simulink library "csu_rtd_translational_dynamics_lib"  (R2014b)
settings: Solver=ode45  SolverMode=SingleTasking  StartTime=0.0  StopTime=10.0  RelTol=1e-3
libraries: util_info_lib x2, util_quat_lib x2, util_integrator_lib x1
settings Model: ExtModeAutoUpdateStatusClock=off  Creator=daniloviazzo  LastModifiedBy=mstewart

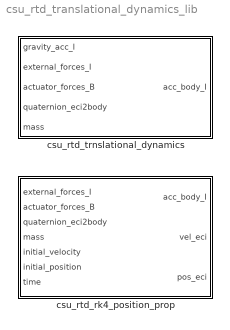
== system csu_rtd_translational_dynamics_lib ==
  csu_rtd_rk4_position_prop : Subsystem
  csu_rtd_trnslational_dynamics : Subsystem

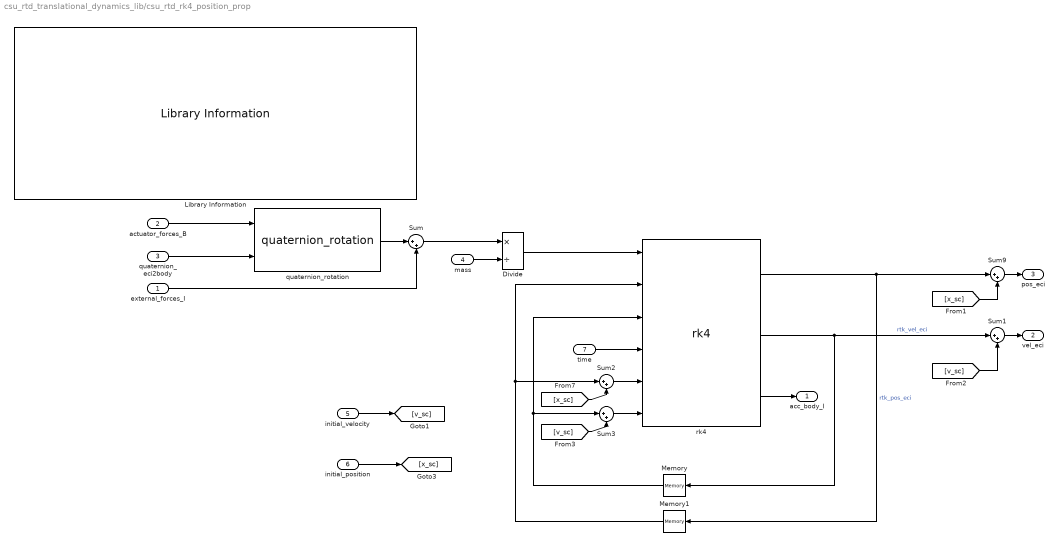
== system csu_rtd_translational_dynamics_lib/csu_rtd_rk4_position_prop ==
  external_forces_I : Inport
  actuator_forces_B : Inport  Port=2
  quaternion_eci2body : Inport  Port=3
  mass : Inport  Port=4
  initial_velocity : Inport  Port=5
  initial_position : Inport  Port=6
  time : Inport  Port=7
  Divide : Product  Inputs=*/
  Library Information : util_info_lib/Library Information  owner='NONE'
  Memory : Memory  InheritSampleTime=on
  Memory1 : Memory  InheritSampleTime=on
  Sum{,1..3,9} (5 alike) : Sum  Inputs=|++
  quaternion_rotation : util_quat_lib/quaternion_rotation  SystemSampleTime=-1
  rk4 : util_integrator_lib/rk4  DT=sim_time_step_size
  acc_body_I : Outport
  vel_eci : Outport  Port=2
  pos_eci : Outport  Port=3
  wires:
  [v_sc] -> Sum3/2
  initial_velocity/1 -> [v_sc]
  [v_sc] -> Sum1/2
  Sum3/1 -> rk4/6
  initial_position/1 -> [x_sc]
  [x_sc] -> Sum2/2
  Sum2/1 -> rk4/5
  [x_sc] -> Sum9/2
  Sum1/1 -> vel_eci/1
  Sum9/1 -> pos_eci/1
  Memory1/1 -> Sum2/1, rk4/2
  Memory/1 -> Sum3/1, rk4/3
  rk4/1 -> Sum9/1, Memory1/1  "rtk_pos_eci"
  time/1 -> rk4/4
  rk4/2 -> Sum1/1, Memory/1  "rtk_vel_eci"
  rk4/3 -> acc_body_I/1
  mass/1 -> Divide/2
  Sum/1 -> Divide/1
  external_forces_I/1 -> Sum/2
  quaternion_rotation/1 -> Sum/1
  quaternion_eci2body/1 -> quaternion_rotation/2
  Divide/1 -> rk4/1
  actuator_forces_B/1 -> quaternion_rotation/1

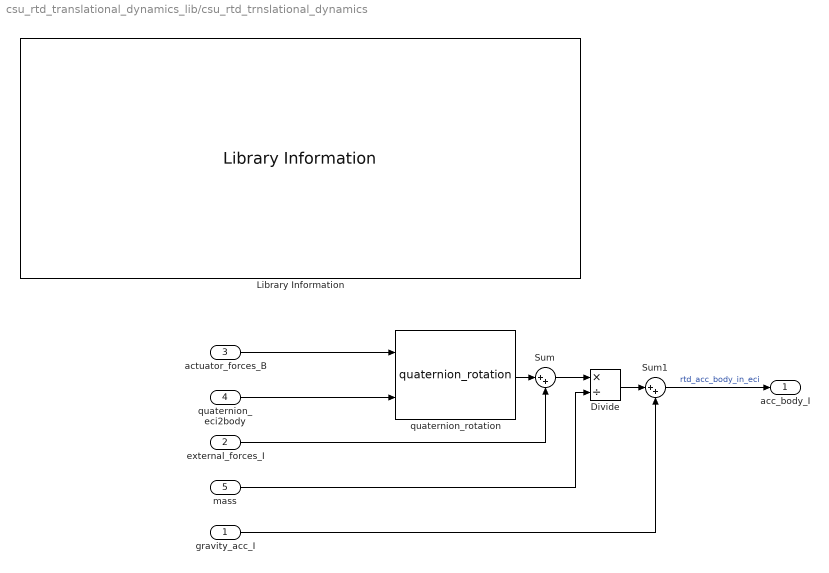
== system csu_rtd_translational_dynamics_lib/csu_rtd_trnslational_dynamics ==
  gravity_acc_I : Inport
  external_forces_I : Inport  Port=2
  actuator_forces_B : Inport  Port=3
  quaternion_eci2body : Inport  Port=4
  mass : Inport  Port=5
  Divide : Product  Inputs=*/
  Library Information : util_info_lib/Library Information  owner='NONE'
  Sum : Sum  Inputs=|++
  Sum1 : Sum  Inputs=|++
  quaternion_rotation : util_quat_lib/quaternion_rotation  SystemSampleTime=-1
  acc_body_I : Outport
  wires:
  Sum1/1 -> acc_body_I/1  "rtd_acc_body_in_eci"
  gravity_acc_I/1 -> Sum1/2
  mass/1 -> Divide/2
  Sum/1 -> Divide/1
  external_forces_I/1 -> Sum/2
  quaternion_rotation/1 -> Sum/1
  quaternion_eci2body/1 -> quaternion_rotation/2
  Divide/1 -> Sum1/1
  actuator_forces_B/1 -> quaternion_rotation/1
